simulink model "Adjoint_MIMO"  (R2017b)
settings: Solver=ode4  StartTime=0.0  StopTime=Tend  FixedStep=Ts  RelTol=1e-3  EnableMultiTasking=on
values from neighbouring files (symbols this model uses):
  A_rc_lat_O = [0 0 0 0 0 0 393.72 0 0 0 0 0 ... (36 elements, 6x6)]    [longlatParameters.mat]
  A_rc_long_O = [0 0 0 0 0 0 0 0 0 0.000111135 2.52e-06 7.98e-12 ... (36 elements, 6x6)]    [longlatParameters.mat]
  Arc = [0 0 0 -3.79740657573 0.00492323855906 0.0757867668346 0 0 0 0 0 0 ... (144 elements, 12x12)]    [longlatParameters.mat]
  B_rc_lat_O = [0  0; 0  0; 0  0; 0.0002  0.0005; -0.3043  0.0583; -0.0126  -0.0293]    [longlatParameters.mat]
  B_rc_long_O = [0  0; 0  0; 0  0; 0.001559526  0.000437475; -4.6e-07  -0.001426346; 0  -0.086580984]    [longlatParameters.mat]
  Brc = [0 0 0 0.4753435248 -0.00046 0 0 0 0 0 0 0 ... (48 elements, 12x4)]    [longlatParameters.mat]
  C_rc_lat_O = [1 0 0 0 0 1 0 0 0 0 1 0 ... (24 elements, 4x6)]    [longlatParameters.mat]
  C_rc_long_O = [1 0 0 0 0 1 0 0 0 0 1 0 ... (24 elements, 4x6)]    [longlatParameters.mat]
  flag_x = 1    [IdealTrack_v3_longlat.m]
  flag_y = 1    [IdealTrack_v3_longlat.m]
  flag_z = 1    [IdealTrack_v3_longlat.m]
  Kp_lat_O = [-2.4334  -1235.6  81.67  -1103.7  -11.02  -64.389; 0.2801  -33.67  -3.4425  -20.635  -1.726  -13.587]    [longlatParameters.mat]
  Kp_long_O = [2.4349  0.2668  53.4474  3.0008  -63.2722  0.1787; 0.2668  -2.434  -886.701  0.2458  667.9862  -77.6272]    [longlatParameters.mat]
libraries: simulink x1
settings Model: Creator=WhisPer  LastModifiedBy=Jinrui
settings DataIOCC: LimitDataPoints=on
settings OptimizationCC: LifeSpan=inf
settings DebuggingCC: AllowSymbolicDim=off  SFUnexpectedBacktrackingDiag=warning  SFNoUnconditionalDefaultTransitionDiag=warning  SFExecutionAtInitializationDiag=none
settings ModelReferenceCC: PropagateSignalLabelsOutOfModel=off
settings CodeAppCC: StateflowObjectComments=on
settings GRTTargetCC: TargetLangStandard=C89/C90 (ANSI)
settings ConfigComp: CovMetricSettings=dw  CovHtmlReporting=on  CovSaveCumulativeToWorkspaceVar=on  CovSaveSingleToWorkspaceVar=on  CovExternalEMLEnable=off

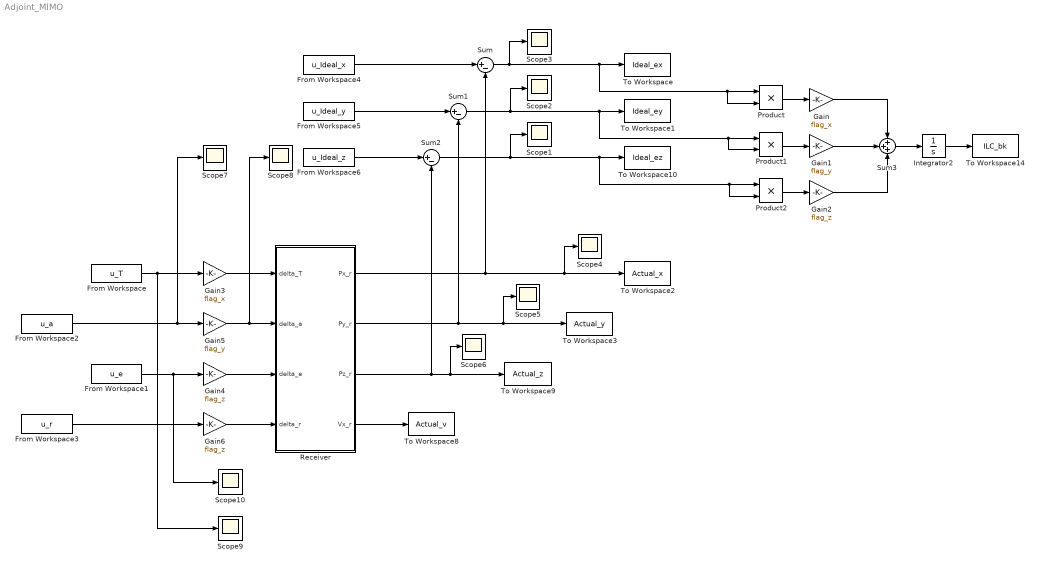
== system Adjoint_MIMO ==
  From Workspace : FromWorkspace  VariableName=u_T  SampleTime=0
  From Workspace1 : FromWorkspace  VariableName=u_e  SampleTime=0
  From Workspace2 : FromWorkspace  VariableName=u_a  SampleTime=0
  From Workspace3 : FromWorkspace  VariableName=u_r  SampleTime=0
  From Workspace4 : FromWorkspace  VariableName=u_Ideal_x  SampleTime=0
  From Workspace5 : FromWorkspace  VariableName=u_Ideal_y  SampleTime=0
  From Workspace6 : FromWorkspace  VariableName=u_Ideal_z  SampleTime=0
  Gain : Gain  Gain=flag_x
  Gain1 : Gain  Gain=flag_y
  Gain2 : Gain  Gain=flag_z
  Gain3 : Gain  Gain=flag_x
  Gain4 : Gain  Gain=flag_z
  Gain5 : Gain  Gain=flag_y
  Gain6 : Gain  Gain=flag_z
  Integrator2 : Integrator
  Product : Product
  Product1 : Product
  Product2 : Product
  Receiver : Subsystem
  Scope{1..10} (10 alike) : Scope
  Sum : Sum  Inputs=|+-
  Sum1 : Sum  Inputs=|+-
  Sum2 : Sum  Inputs=|+-
  Sum3 : Sum  Inputs=+++
  To Workspace : ToWorkspace  VariableName=Ideal_ex  SampleTime=-1
  To Workspace1 : ToWorkspace  VariableName=Ideal_ey  SampleTime=-1
  To Workspace10 : ToWorkspace  VariableName=Ideal_ez  SampleTime=-1
  To Workspace14 : ToWorkspace  VariableName=ILC_bk  SampleTime=-1
  To Workspace2 : ToWorkspace  VariableName=Actual_x  SampleTime=-1
  To Workspace3 : ToWorkspace  VariableName=Actual_y  SampleTime=-1
  To Workspace8 : ToWorkspace  VariableName=Actual_v  SampleTime=-1
  To Workspace9 : ToWorkspace  VariableName=Actual_z  SampleTime=-1
  wires:
  From Workspace/1 -> Scope9/1, Gain3/1
  From Workspace1/1 -> Scope10/1, Gain4/1
  From Workspace4/1 -> Sum/1
  From Workspace5/1 -> Sum1/1
  Sum/1 -> Scope3/1, Product/2, Product/1, To Workspace/1
  Sum1/1 -> Scope2/1, Product1/2, Product1/1, To Workspace1/1
  Receiver/4(Vx_r) -> To Workspace8/1
  From Workspace6/1 -> Sum2/1
  Sum2/1 -> Scope1/1, Product2/2, Product2/1, To Workspace10/1
  From Workspace2/1 -> Scope7/1, Gain5/1
  From Workspace3/1 -> Gain6/1
  Receiver/1(Px_r) -> Scope4/1, To Workspace2/1, Sum/2
  Product/1 -> Gain/1
  Receiver/2(Py_r) -> Scope5/1, To Workspace3/1, Sum1/2
  Receiver/3(Pz_r) -> Scope6/1, To Workspace9/1, Sum2/2
  Sum3/1 -> Integrator2/1
  Integrator2/1 -> To Workspace14/1
  Product1/1 -> Gain1/1
  Product2/1 -> Gain2/1
  Gain/1 -> Sum3/1
  Gain1/1 -> Sum3/2
  Gain2/1 -> Sum3/3
  Gain3/1 -> Receiver/1(delta_T)
  Gain5/1 -> Scope8/1, Receiver/2(delta_a)
  Gain4/1 -> Receiver/3(delta_e)
  Gain6/1 -> Receiver/4(delta_r)

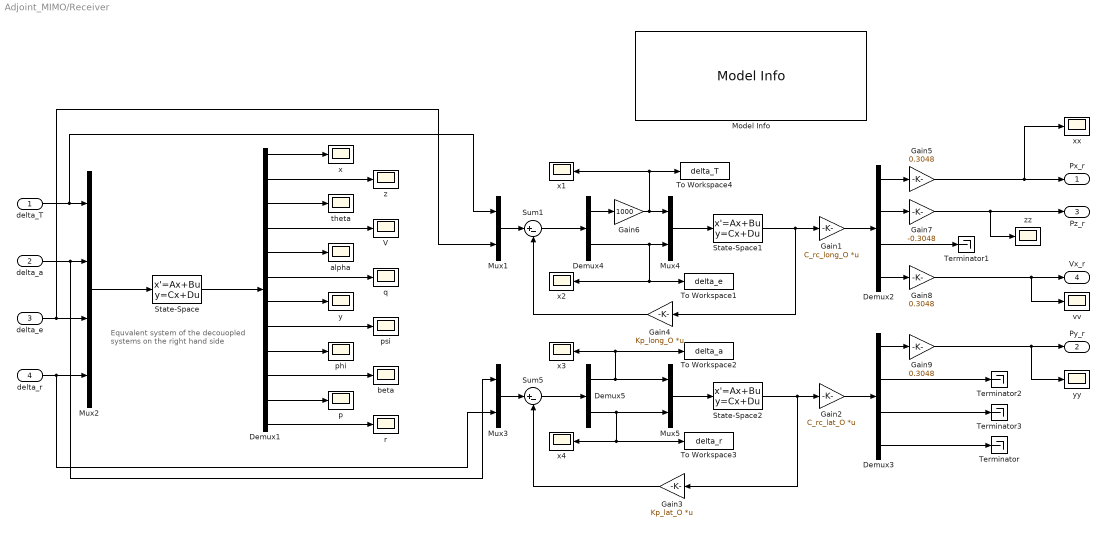
== system Adjoint_MIMO/Receiver ==
  note: Equvalent system of the decouopled
      | systems on the right hand side
  delta_T : Inport
  delta_a : Inport  Port=2
  delta_e : Inport  Port=3
  delta_r : Inport  Port=4
  Demux1 : Demux  Outputs=12
  Demux2 : Demux
  Demux3 : Demux
  Demux4 : Demux  Outputs=2
  Demux5 : Demux  Outputs=2
  Gain1 : Gain  Gain=C_rc_long_O  Multiplication=Matrix(K*u) (u vector)
  Gain2 : Gain  Gain=C_rc_lat_O  Multiplication=Matrix(K*u) (u vector)
  Gain3 : Gain  Gain=Kp_lat_O  Multiplication=Matrix(K*u) (u vector)
  Gain4 : Gain  Gain=Kp_long_O  Multiplication=Matrix(K*u) (u vector)
  Gain5 : Gain  Gain=0.3048
  Gain6 : Gain  Gain=1000
  Gain7 : Gain  Gain=-0.3048
  Gain8 : Gain  Gain=0.3048
  Gain9 : Gain  Gain=0.3048
  Model Info : simulink/Model-Wide Utilities/Model Info  Frame=on  DisplayStringWithTags=delta_e + => pitch - => h -  HorizontalTextAlignment=Center  LeftAlignmentValue=0.5
  Mux{1,3..5} (4 alike) : Mux  Inputs=2
  Mux2 : Mux
  State-Space : StateSpace  A=Arc  B=Brc  C=eye(size(Arc,1),size(Arc,1))  D=zeros(size(Arc,1),size(Brc,2))  InitialCondition=0
  State-Space1 : StateSpace  A=A_rc_long_O  B=B_rc_long_O  C=eye(6,6)  D=zeros(6,2)  InitialCondition=0
  State-Space2 : StateSpace  A=A_rc_lat_O  B=B_rc_lat_O  C=eye(6,6)  D=zeros(6,2)  InitialCondition=0
  Sum1 : Sum  Inputs=|+-
  Sum5 : Sum  Inputs=|+-
  Terminator{,1..3} (4 alike) : Terminator
  To Workspace1 : ToWorkspace  VariableName=delta_e  SampleTime=-1
  To Workspace2 : ToWorkspace  VariableName=delta_a  SampleTime=-1
  To Workspace3 : ToWorkspace  VariableName=delta_r  SampleTime=-1
  To Workspace4 : ToWorkspace  VariableName=delta_T  SampleTime=-1
  V : Scope
  alpha : Scope
  beta : Scope
  p : Scope
  phi : Scope
  psi : Scope
  q : Scope
  r : Scope
  theta : Scope
  vv : Scope
  x{,1..4} (5 alike) : Scope
  xx : Scope
  y : Scope
  yy : Scope
  z : Scope
  zz : Scope
  Px_r : Outport
  Py_r : Outport  Port=2
  Pz_r : Outport  Port=3
  Vx_r : Outport  Port=4
  wires:
  Mux2/1 -> State-Space/1
  State-Space/1 -> Demux1/1
  Demux1/1 -> x/1
  Demux1/2 -> z/1
  Demux1/3 -> theta/1
  Demux1/4 -> V/1
  Demux1/5 -> alpha/1
  Demux1/6 -> q/1
  Demux1/7 -> y/1
  Demux1/8 -> psi/1
  Demux1/9 -> phi/1
  Demux1/10 -> beta/1
  Demux1/11 -> p/1
  Demux1/12 -> r/1
  Sum1/1 -> Demux4/1
  Demux4/2 -> x2/1, To Workspace1/1, Mux4/2
  Demux4/1 -> Gain6/1
  Gain6/1 -> To Workspace4/1, x1/1, Mux4/1
  Mux4/1 -> State-Space1/1
  State-Space1/1 -> Gain4/1, Gain1/1
  Gain4/1 -> Sum1/2
  Mux1/1 -> Sum1/1
  Gain1/1 -> Demux2/1
  delta_T/1 -> Mux1/1, Mux2/1
  delta_e/1 -> Mux1/2, Mux2/3
  Demux2/3 -> Terminator1/1
  Demux2/4 -> Gain8/1
  Demux2/1 -> Gain5/1
  Demux2/2 -> Gain7/1
  State-Space2/1 -> Gain3/1, Gain2/1
  Gain3/1 -> Sum5/2
  Mux3/1 -> Sum5/1
  delta_a/1 -> Mux3/1, Mux2/2
  delta_r/1 -> Mux3/2, Mux2/4
  Gain2/1 -> Demux3/1
  Demux3/4 -> Terminator/1
  Demux3/1 -> Gain9/1
  Gain5/1 -> xx/1, Px_r/1
  Gain7/1 -> Pz_r/1, zz/1
  Gain8/1 -> vv/1, Vx_r/1
  Gain9/1 -> yy/1, Py_r/1
  Demux3/2 -> Terminator2/1
  Demux3/3 -> Terminator3/1
  Sum5/1 -> Demux5/1
  Demux5/2 -> x4/1, To Workspace3/1, Mux5/2
  Demux5/1 -> x3/1, To Workspace2/1, Mux5/1
  Mux5/1 -> State-Space2/1
